simulink model "teste2"  (R2018a)
settings: Solver=VariableStepAuto  StartTime=0.0  StopTime=20  RelTol=1e-9
libraries: arduino_io_lib x5
settings Model: Creator=Mauricio  LastModifiedBy=Mauricio

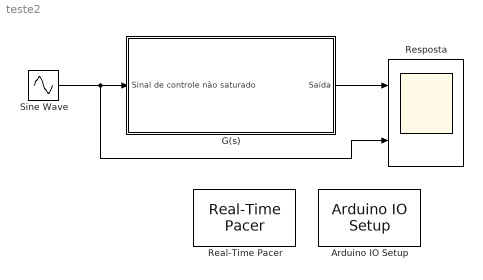
== system teste2 ==
  Arduino IO Setup : arduino_io_lib/Arduino IO Setup  Priority=3  arduinoVar=Temporary arduino variable: Arduino1  workspaceVarName=a  comPort=COM6
  "G(s) " : Subsystem
  Real-Time Pacer : arduino_io_lib/Real-Time Pacer  simTimePerRealTime=1
  Resposta : Scope  NumInputPorts=2
  Sine Wave : Sin  Amplitude=200  Frequency=3
  wires:
  "G(s) "/1(Saída) -> Resposta/1
  Sine Wave/1 -> Resposta/2, "G(s) "/1(Sinal de controle não saturado)

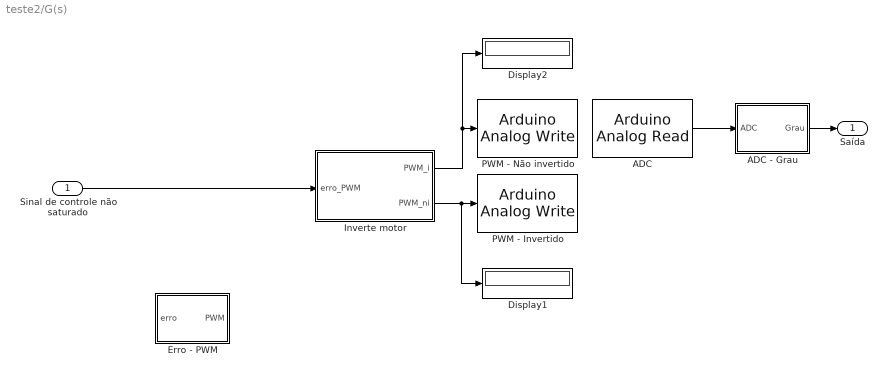
== system teste2/G(s)  ==
  Sinal de controle não saturado : Inport
  ADC : arduino_io_lib/Arduino Analog Read  arduinoVar=Temporary arduino variable: Arduino1  arduinoPin=2  T=0.025
  ADC - Grau : MATLAB Function  TreatAsAtomicUnit=on
  Display1 : Display
  Display2 : Display
  Erro - PWM : MATLAB Function  TreatAsAtomicUnit=on
  Inverte motor : MATLAB Function  TreatAsAtomicUnit=on
  PWM - Invertido : arduino_io_lib/Arduino Analog Write  arduinoVar=Temporary arduino variable: Arduino1  arduinoPin=6  T=0.025
  PWM - Não invertido : arduino_io_lib/Arduino Analog Write  arduinoVar=Temporary arduino variable: Arduino1  arduinoPin=5  T=0.025
  Saída : Outport
  wires:
  ADC/1 -> ADC - Grau/1(ADC)
  Inverte motor/2(PWM_ni) -> Display1/1, PWM - Invertido/1
  Inverte motor/1(PWM_i) -> Display2/1, PWM - Não invertido/1
  ADC - Grau/1(Grau) -> Saída/1
  Sinal de controle não saturado/1 -> Inverte motor/1(erro_PWM)

== matlab function teste2/G(s) /Erro - PWM ==
  data: erro input; PWM output
function PWM = fcn(erro)

if(erro < pi/180 && erro >=0)
    PWM = 0;
elseif(erro > -pi/180 && erro < 0)
    PWM = 0;
else
    PWM = 150.7783671396903180968372495108*erro + 57.368421052631578947368421052632;
end

== matlab function teste2/G(s) /ADC - Grau ==
  data: ADC input; Grau output
function Grau = fcn(ADC)
Grau = -0.17413322126497163269594452616096*ADC + 136.2690584156335364572389157386;

== matlab function teste2/G(s) /Inverte motor ==
  data: PWM_i output; PWM_ni output; erro_PWM input
function [PWM_i, PWM_ni] = fcn(erro_PWM)

%REVERSO
if(erro_PWM>0)
    PWM_i = erro_PWM;
    PWM_ni = 0;
%FRENTE
elseif(erro_PWM<0)
    PWM_ni = abs(erro_PWM);
    PWM_i = 0;
%DESLIGADO
else
    PWM_ni = 0;
    PWM_i = 0;
end
